simulink model "gm_hybrid_lht"  (R2019b)
settings: Solver=FixedStepDiscrete  StartTime=0.0  StopTime=inf  FixedStep=1/120e6  RelTol=1e-3
undefined symbols (not defined in the file or in its folder): bt, height, nTheta, width
libraries: hdlsllib x237, simulink x149, hdlmdlgenlib x11, dspsrcs4 x1
(part 6 of 11)

== system gm_hybrid_lht/Hybrid LHT/Hybrid LHT Accumulator/Accumulator with Switches/Accumulator_instance10/Block RAM ==
  wr_data : Inport  OutDataTypeStr=fixdt(0, 36, 0)  PortDimensions=1  SampleTime=8.33333333333333e-09
  wr_addr : Inport  Port=2  OutDataTypeStr=fixdt(0, 9, 0)  PortDimensions=1  SampleTime=8.33333333333333e-09
  wr_en : Inport  Port=3  OutDataTypeStr=boolean  PortDimensions=1  SampleTime=8.33333333333333e-09
  rd_addr : Inport  Port=4  OutDataTypeStr=fixdt(0, 9, 0)  PortDimensions=1  SampleTime=8.33333333333333e-09
  Simple Dual Port RAM Generator : Subsystem  mask{b=double(36), d=double(400), b_hidden=double(36), d_hidden=double(400)}
      mask prompts: b "Data width:"; d "Depth:"
      mask init: same as gm_hybrid_lht/Hybrid LHT/Hybrid LHT Accumulator/Accumulator with Switches/Accumulator_instance1/Block RAM/Simple Dual Port RAM Generator
  rd_data : Outport
  wires:
  rd_addr/1 -> Simple Dual Port RAM Generator/4(rd_addr)
  wr_en/1 -> Simple Dual Port RAM Generator/3(wr_en)
  wr_addr/1 -> Simple Dual Port RAM Generator/2(wr_addr)
  wr_data/1 -> Simple Dual Port RAM Generator/1(wr_data)
  Simple Dual Port RAM Generator/1(rd_data) -> rd_data/1

== system gm_hybrid_lht/Hybrid LHT/Hybrid LHT Accumulator/Accumulator with Switches/Accumulator_instance11/Block RAM ==
  wr_data : Inport  OutDataTypeStr=fixdt(0, 36, 0)  PortDimensions=1  SampleTime=8.33333333333333e-09
  wr_addr : Inport  Port=2  OutDataTypeStr=fixdt(0, 9, 0)  PortDimensions=1  SampleTime=8.33333333333333e-09
  wr_en : Inport  Port=3  OutDataTypeStr=boolean  PortDimensions=1  SampleTime=8.33333333333333e-09
  rd_addr : Inport  Port=4  OutDataTypeStr=fixdt(0, 9, 0)  PortDimensions=1  SampleTime=8.33333333333333e-09
  Simple Dual Port RAM Generator : Subsystem  mask{b=double(36), d=double(400), b_hidden=double(36), d_hidden=double(400)}
      mask prompts: b "Data width:"; d "Depth:"
      mask init: same as gm_hybrid_lht/Hybrid LHT/Hybrid LHT Accumulator/Accumulator with Switches/Accumulator_instance1/Block RAM/Simple Dual Port RAM Generator
  rd_data : Outport
  wires:
  rd_addr/1 -> Simple Dual Port RAM Generator/4(rd_addr)
  wr_en/1 -> Simple Dual Port RAM Generator/3(wr_en)
  wr_addr/1 -> Simple Dual Port RAM Generator/2(wr_addr)
  wr_data/1 -> Simple Dual Port RAM Generator/1(wr_data)
  Simple Dual Port RAM Generator/1(rd_data) -> rd_data/1

== system gm_hybrid_lht/Hybrid LHT/Hybrid LHT Accumulator/Accumulator with Switches/Accumulator_instance12/Block RAM ==
  wr_data : Inport  OutDataTypeStr=fixdt(0, 36, 0)  PortDimensions=1  SampleTime=8.33333333333333e-09
  wr_addr : Inport  Port=2  OutDataTypeStr=fixdt(0, 9, 0)  PortDimensions=1  SampleTime=8.33333333333333e-09
  wr_en : Inport  Port=3  OutDataTypeStr=boolean  PortDimensions=1  SampleTime=8.33333333333333e-09
  rd_addr : Inport  Port=4  OutDataTypeStr=fixdt(0, 9, 0)  PortDimensions=1  SampleTime=8.33333333333333e-09
  Simple Dual Port RAM Generator : Subsystem  mask{b=double(36), d=double(400), b_hidden=double(36), d_hidden=double(400)}
      mask prompts: b "Data width:"; d "Depth:"
      mask init: same as gm_hybrid_lht/Hybrid LHT/Hybrid LHT Accumulator/Accumulator with Switches/Accumulator_instance1/Block RAM/Simple Dual Port RAM Generator
  rd_data : Outport
  wires:
  rd_addr/1 -> Simple Dual Port RAM Generator/4(rd_addr)
  wr_en/1 -> Simple Dual Port RAM Generator/3(wr_en)
  wr_addr/1 -> Simple Dual Port RAM Generator/2(wr_addr)
  wr_data/1 -> Simple Dual Port RAM Generator/1(wr_data)
  Simple Dual Port RAM Generator/1(rd_data) -> rd_data/1

== system gm_hybrid_lht/Hybrid LHT/Hybrid LHT Accumulator/Accumulator with Switches/Accumulator_instance13/Block RAM ==
  wr_data : Inport  OutDataTypeStr=fixdt(0, 36, 0)  PortDimensions=1  SampleTime=8.33333333333333e-09
  wr_addr : Inport  Port=2  OutDataTypeStr=fixdt(0, 9, 0)  PortDimensions=1  SampleTime=8.33333333333333e-09
  wr_en : Inport  Port=3  OutDataTypeStr=boolean  PortDimensions=1  SampleTime=8.33333333333333e-09
  rd_addr : Inport  Port=4  OutDataTypeStr=fixdt(0, 9, 0)  PortDimensions=1  SampleTime=8.33333333333333e-09
  Simple Dual Port RAM Generator : Subsystem  mask{b=double(36), d=double(400), b_hidden=double(36), d_hidden=double(400)}
      mask prompts: b "Data width:"; d "Depth:"
      mask init: same as gm_hybrid_lht/Hybrid LHT/Hybrid LHT Accumulator/Accumulator with Switches/Accumulator_instance1/Block RAM/Simple Dual Port RAM Generator
  rd_data : Outport
  wires:
  rd_addr/1 -> Simple Dual Port RAM Generator/4(rd_addr)
  wr_en/1 -> Simple Dual Port RAM Generator/3(wr_en)
  wr_addr/1 -> Simple Dual Port RAM Generator/2(wr_addr)
  wr_data/1 -> Simple Dual Port RAM Generator/1(wr_data)
  Simple Dual Port RAM Generator/1(rd_data) -> rd_data/1

== system gm_hybrid_lht/Hybrid LHT/Hybrid LHT Accumulator/Accumulator with Switches/Accumulator_instance14/Block RAM ==
  wr_data : Inport  OutDataTypeStr=fixdt(0, 36, 0)  PortDimensions=1  SampleTime=8.33333333333333e-09
  wr_addr : Inport  Port=2  OutDataTypeStr=fixdt(0, 9, 0)  PortDimensions=1  SampleTime=8.33333333333333e-09
  wr_en : Inport  Port=3  OutDataTypeStr=boolean  PortDimensions=1  SampleTime=8.33333333333333e-09
  rd_addr : Inport  Port=4  OutDataTypeStr=fixdt(0, 9, 0)  PortDimensions=1  SampleTime=8.33333333333333e-09
  Simple Dual Port RAM Generator : Subsystem  mask{b=double(36), d=double(400), b_hidden=double(36), d_hidden=double(400)}
      mask prompts: b "Data width:"; d "Depth:"
      mask init: same as gm_hybrid_lht/Hybrid LHT/Hybrid LHT Accumulator/Accumulator with Switches/Accumulator_instance1/Block RAM/Simple Dual Port RAM Generator
  rd_data : Outport
  wires:
  rd_addr/1 -> Simple Dual Port RAM Generator/4(rd_addr)
  wr_en/1 -> Simple Dual Port RAM Generator/3(wr_en)
  wr_addr/1 -> Simple Dual Port RAM Generator/2(wr_addr)
  wr_data/1 -> Simple Dual Port RAM Generator/1(wr_data)
  Simple Dual Port RAM Generator/1(rd_data) -> rd_data/1

== system gm_hybrid_lht/Hybrid LHT/Hybrid LHT Accumulator/Accumulator with Switches/Accumulator_instance15/Block RAM ==
  wr_data : Inport  OutDataTypeStr=fixdt(0, 36, 0)  PortDimensions=1  SampleTime=8.33333333333333e-09
  wr_addr : Inport  Port=2  OutDataTypeStr=fixdt(0, 9, 0)  PortDimensions=1  SampleTime=8.33333333333333e-09
  wr_en : Inport  Port=3  OutDataTypeStr=boolean  PortDimensions=1  SampleTime=8.33333333333333e-09
  rd_addr : Inport  Port=4  OutDataTypeStr=fixdt(0, 9, 0)  PortDimensions=1  SampleTime=8.33333333333333e-09
  Simple Dual Port RAM Generator : Subsystem  mask{b=double(36), d=double(400), b_hidden=double(36), d_hidden=double(400)}
      mask prompts: b "Data width:"; d "Depth:"
      mask init: same as gm_hybrid_lht/Hybrid LHT/Hybrid LHT Accumulator/Accumulator with Switches/Accumulator_instance1/Block RAM/Simple Dual Port RAM Generator
  rd_data : Outport
  wires:
  rd_addr/1 -> Simple Dual Port RAM Generator/4(rd_addr)
  wr_en/1 -> Simple Dual Port RAM Generator/3(wr_en)
  wr_addr/1 -> Simple Dual Port RAM Generator/2(wr_addr)
  wr_data/1 -> Simple Dual Port RAM Generator/1(wr_data)
  Simple Dual Port RAM Generator/1(rd_data) -> rd_data/1

== system gm_hybrid_lht/Hybrid LHT/Hybrid LHT Accumulator/Accumulator with Switches/Accumulator_instance16/Block RAM ==
  wr_data : Inport  OutDataTypeStr=fixdt(0, 36, 0)  PortDimensions=1  SampleTime=8.33333333333333e-09
  wr_addr : Inport  Port=2  OutDataTypeStr=fixdt(0, 9, 0)  PortDimensions=1  SampleTime=8.33333333333333e-09
  wr_en : Inport  Port=3  OutDataTypeStr=boolean  PortDimensions=1  SampleTime=8.33333333333333e-09
  rd_addr : Inport  Port=4  OutDataTypeStr=fixdt(0, 9, 0)  PortDimensions=1  SampleTime=8.33333333333333e-09
  Simple Dual Port RAM Generator : Subsystem  mask{b=double(36), d=double(400), b_hidden=double(36), d_hidden=double(400)}
      mask prompts: b "Data width:"; d "Depth:"
      mask init: same as gm_hybrid_lht/Hybrid LHT/Hybrid LHT Accumulator/Accumulator with Switches/Accumulator_instance1/Block RAM/Simple Dual Port RAM Generator
  rd_data : Outport
  wires:
  rd_addr/1 -> Simple Dual Port RAM Generator/4(rd_addr)
  wr_en/1 -> Simple Dual Port RAM Generator/3(wr_en)
  wr_addr/1 -> Simple Dual Port RAM Generator/2(wr_addr)
  wr_data/1 -> Simple Dual Port RAM Generator/1(wr_data)
  Simple Dual Port RAM Generator/1(rd_data) -> rd_data/1

== system gm_hybrid_lht/Hybrid LHT/Hybrid LHT Accumulator/Accumulator with Switches/Accumulator_instance17/Block RAM ==
  wr_data : Inport  OutDataTypeStr=fixdt(0, 36, 0)  PortDimensions=1  SampleTime=8.33333333333333e-09
  wr_addr : Inport  Port=2  OutDataTypeStr=fixdt(0, 9, 0)  PortDimensions=1  SampleTime=8.33333333333333e-09
  wr_en : Inport  Port=3  OutDataTypeStr=boolean  PortDimensions=1  SampleTime=8.33333333333333e-09
  rd_addr : Inport  Port=4  OutDataTypeStr=fixdt(0, 9, 0)  PortDimensions=1  SampleTime=8.33333333333333e-09
  Simple Dual Port RAM Generator : Subsystem  mask{b=double(36), d=double(400), b_hidden=double(36), d_hidden=double(400)}
      mask prompts: b "Data width:"; d "Depth:"
      mask init: same as gm_hybrid_lht/Hybrid LHT/Hybrid LHT Accumulator/Accumulator with Switches/Accumulator_instance1/Block RAM/Simple Dual Port RAM Generator
  rd_data : Outport
  wires:
  rd_addr/1 -> Simple Dual Port RAM Generator/4(rd_addr)
  wr_en/1 -> Simple Dual Port RAM Generator/3(wr_en)
  wr_addr/1 -> Simple Dual Port RAM Generator/2(wr_addr)
  wr_data/1 -> Simple Dual Port RAM Generator/1(wr_data)
  Simple Dual Port RAM Generator/1(rd_data) -> rd_data/1

== system gm_hybrid_lht/Hybrid LHT/Hybrid LHT Accumulator/Accumulator with Switches/Accumulator_instance18/Block RAM ==
  wr_data : Inport  OutDataTypeStr=fixdt(0, 36, 0)  PortDimensions=1  SampleTime=8.33333333333333e-09
  wr_addr : Inport  Port=2  OutDataTypeStr=fixdt(0, 9, 0)  PortDimensions=1  SampleTime=8.33333333333333e-09
  wr_en : Inport  Port=3  OutDataTypeStr=boolean  PortDimensions=1  SampleTime=8.33333333333333e-09
  rd_addr : Inport  Port=4  OutDataTypeStr=fixdt(0, 9, 0)  PortDimensions=1  SampleTime=8.33333333333333e-09
  Simple Dual Port RAM Generator : Subsystem  mask{b=double(36), d=double(400), b_hidden=double(36), d_hidden=double(400)}
      mask prompts: b "Data width:"; d "Depth:"
      mask init: same as gm_hybrid_lht/Hybrid LHT/Hybrid LHT Accumulator/Accumulator with Switches/Accumulator_instance1/Block RAM/Simple Dual Port RAM Generator
  rd_data : Outport
  wires:
  rd_addr/1 -> Simple Dual Port RAM Generator/4(rd_addr)
  wr_en/1 -> Simple Dual Port RAM Generator/3(wr_en)
  wr_addr/1 -> Simple Dual Port RAM Generator/2(wr_addr)
  wr_data/1 -> Simple Dual Port RAM Generator/1(wr_data)
  Simple Dual Port RAM Generator/1(rd_data) -> rd_data/1

== system gm_hybrid_lht/Hybrid LHT/Hybrid LHT Accumulator/Accumulator with Switches/Accumulator_instance19/Block RAM ==
  wr_data : Inport  OutDataTypeStr=fixdt(0, 36, 0)  PortDimensions=1  SampleTime=8.33333333333333e-09
  wr_addr : Inport  Port=2  OutDataTypeStr=fixdt(0, 9, 0)  PortDimensions=1  SampleTime=8.33333333333333e-09
  wr_en : Inport  Port=3  OutDataTypeStr=boolean  PortDimensions=1  SampleTime=8.33333333333333e-09
  rd_addr : Inport  Port=4  OutDataTypeStr=fixdt(0, 9, 0)  PortDimensions=1  SampleTime=8.33333333333333e-09
  Simple Dual Port RAM Generator : Subsystem  mask{b=double(36), d=double(400), b_hidden=double(36), d_hidden=double(400)}
      mask prompts: b "Data width:"; d "Depth:"
      mask init: same as gm_hybrid_lht/Hybrid LHT/Hybrid LHT Accumulator/Accumulator with Switches/Accumulator_instance1/Block RAM/Simple Dual Port RAM Generator
  rd_data : Outport
  wires:
  rd_addr/1 -> Simple Dual Port RAM Generator/4(rd_addr)
  wr_en/1 -> Simple Dual Port RAM Generator/3(wr_en)
  wr_addr/1 -> Simple Dual Port RAM Generator/2(wr_addr)
  wr_data/1 -> Simple Dual Port RAM Generator/1(wr_data)
  Simple Dual Port RAM Generator/1(rd_data) -> rd_data/1

== system gm_hybrid_lht/Hybrid LHT/Hybrid LHT Accumulator/Accumulator with Switches/Accumulator_instance2/Block RAM ==
  wr_data : Inport  OutDataTypeStr=fixdt(0, 36, 0)  PortDimensions=1  SampleTime=8.33333333333333e-09
  wr_addr : Inport  Port=2  OutDataTypeStr=fixdt(0, 9, 0)  PortDimensions=1  SampleTime=8.33333333333333e-09
  wr_en : Inport  Port=3  OutDataTypeStr=boolean  PortDimensions=1  SampleTime=8.33333333333333e-09
  rd_addr : Inport  Port=4  OutDataTypeStr=fixdt(0, 9, 0)  PortDimensions=1  SampleTime=8.33333333333333e-09
  Simple Dual Port RAM Generator : Subsystem  mask{b=double(36), d=double(400), b_hidden=double(36), d_hidden=double(400)}
      mask prompts: b "Data width:"; d "Depth:"
      mask init: same as gm_hybrid_lht/Hybrid LHT/Hybrid LHT Accumulator/Accumulator with Switches/Accumulator_instance1/Block RAM/Simple Dual Port RAM Generator
  rd_data : Outport
  wires:
  rd_addr/1 -> Simple Dual Port RAM Generator/4(rd_addr)
  wr_en/1 -> Simple Dual Port RAM Generator/3(wr_en)
  wr_addr/1 -> Simple Dual Port RAM Generator/2(wr_addr)
  wr_data/1 -> Simple Dual Port RAM Generator/1(wr_data)
  Simple Dual Port RAM Generator/1(rd_data) -> rd_data/1

== system gm_hybrid_lht/Hybrid LHT/Hybrid LHT Accumulator/Accumulator with Switches/Accumulator_instance20/Block RAM ==
  wr_data : Inport  OutDataTypeStr=fixdt(0, 36, 0)  PortDimensions=1  SampleTime=8.33333333333333e-09
  wr_addr : Inport  Port=2  OutDataTypeStr=fixdt(0, 9, 0)  PortDimensions=1  SampleTime=8.33333333333333e-09
  wr_en : Inport  Port=3  OutDataTypeStr=boolean  PortDimensions=1  SampleTime=8.33333333333333e-09
  rd_addr : Inport  Port=4  OutDataTypeStr=fixdt(0, 9, 0)  PortDimensions=1  SampleTime=8.33333333333333e-09
  Simple Dual Port RAM Generator : Subsystem  mask{b=double(36), d=double(400), b_hidden=double(36), d_hidden=double(400)}
      mask prompts: b "Data width:"; d "Depth:"
      mask init: same as gm_hybrid_lht/Hybrid LHT/Hybrid LHT Accumulator/Accumulator with Switches/Accumulator_instance1/Block RAM/Simple Dual Port RAM Generator
  rd_data : Outport
  wires:
  rd_addr/1 -> Simple Dual Port RAM Generator/4(rd_addr)
  wr_en/1 -> Simple Dual Port RAM Generator/3(wr_en)
  wr_addr/1 -> Simple Dual Port RAM Generator/2(wr_addr)
  wr_data/1 -> Simple Dual Port RAM Generator/1(wr_data)
  Simple Dual Port RAM Generator/1(rd_data) -> rd_data/1

== system gm_hybrid_lht/Hybrid LHT/Hybrid LHT Accumulator/Accumulator with Switches/Accumulator_instance21/Block RAM ==
  wr_data : Inport  OutDataTypeStr=fixdt(0, 36, 0)  PortDimensions=1  SampleTime=8.33333333333333e-09
  wr_addr : Inport  Port=2  OutDataTypeStr=fixdt(0, 9, 0)  PortDimensions=1  SampleTime=8.33333333333333e-09
  wr_en : Inport  Port=3  OutDataTypeStr=boolean  PortDimensions=1  SampleTime=8.33333333333333e-09
  rd_addr : Inport  Port=4  OutDataTypeStr=fixdt(0, 9, 0)  PortDimensions=1  SampleTime=8.33333333333333e-09
  Simple Dual Port RAM Generator : Subsystem  mask{b=double(36), d=double(400), b_hidden=double(36), d_hidden=double(400)}
      mask prompts: b "Data width:"; d "Depth:"
      mask init: same as gm_hybrid_lht/Hybrid LHT/Hybrid LHT Accumulator/Accumulator with Switches/Accumulator_instance1/Block RAM/Simple Dual Port RAM Generator
  rd_data : Outport
  wires:
  rd_addr/1 -> Simple Dual Port RAM Generator/4(rd_addr)
  wr_en/1 -> Simple Dual Port RAM Generator/3(wr_en)
  wr_addr/1 -> Simple Dual Port RAM Generator/2(wr_addr)
  wr_data/1 -> Simple Dual Port RAM Generator/1(wr_data)
  Simple Dual Port RAM Generator/1(rd_data) -> rd_data/1

== system gm_hybrid_lht/Hybrid LHT/Hybrid LHT Accumulator/Accumulator with Switches/Accumulator_instance22/Block RAM ==
  wr_data : Inport  OutDataTypeStr=fixdt(0, 36, 0)  PortDimensions=1  SampleTime=8.33333333333333e-09
  wr_addr : Inport  Port=2  OutDataTypeStr=fixdt(0, 9, 0)  PortDimensions=1  SampleTime=8.33333333333333e-09
  wr_en : Inport  Port=3  OutDataTypeStr=boolean  PortDimensions=1  SampleTime=8.33333333333333e-09
  rd_addr : Inport  Port=4  OutDataTypeStr=fixdt(0, 9, 0)  PortDimensions=1  SampleTime=8.33333333333333e-09
  Simple Dual Port RAM Generator : Subsystem  mask{b=double(36), d=double(400), b_hidden=double(36), d_hidden=double(400)}
      mask prompts: b "Data width:"; d "Depth:"
      mask init: same as gm_hybrid_lht/Hybrid LHT/Hybrid LHT Accumulator/Accumulator with Switches/Accumulator_instance1/Block RAM/Simple Dual Port RAM Generator
  rd_data : Outport
  wires:
  rd_addr/1 -> Simple Dual Port RAM Generator/4(rd_addr)
  wr_en/1 -> Simple Dual Port RAM Generator/3(wr_en)
  wr_addr/1 -> Simple Dual Port RAM Generator/2(wr_addr)
  wr_data/1 -> Simple Dual Port RAM Generator/1(wr_data)
  Simple Dual Port RAM Generator/1(rd_data) -> rd_data/1

== system gm_hybrid_lht/Hybrid LHT/Hybrid LHT Accumulator/Accumulator with Switches/Accumulator_instance23/Block RAM ==
  wr_data : Inport  OutDataTypeStr=fixdt(0, 36, 0)  PortDimensions=1  SampleTime=8.33333333333333e-09
  wr_addr : Inport  Port=2  OutDataTypeStr=fixdt(0, 9, 0)  PortDimensions=1  SampleTime=8.33333333333333e-09
  wr_en : Inport  Port=3  OutDataTypeStr=boolean  PortDimensions=1  SampleTime=8.33333333333333e-09
  rd_addr : Inport  Port=4  OutDataTypeStr=fixdt(0, 9, 0)  PortDimensions=1  SampleTime=8.33333333333333e-09
  Simple Dual Port RAM Generator : Subsystem  mask{b=double(36), d=double(400), b_hidden=double(36), d_hidden=double(400)}
      mask prompts: b "Data width:"; d "Depth:"
      mask init: same as gm_hybrid_lht/Hybrid LHT/Hybrid LHT Accumulator/Accumulator with Switches/Accumulator_instance1/Block RAM/Simple Dual Port RAM Generator
  rd_data : Outport
  wires:
  rd_addr/1 -> Simple Dual Port RAM Generator/4(rd_addr)
  wr_en/1 -> Simple Dual Port RAM Generator/3(wr_en)
  wr_addr/1 -> Simple Dual Port RAM Generator/2(wr_addr)
  wr_data/1 -> Simple Dual Port RAM Generator/1(wr_data)
  Simple Dual Port RAM Generator/1(rd_data) -> rd_data/1

== system gm_hybrid_lht/Hybrid LHT/Hybrid LHT Accumulator/Accumulator with Switches/Accumulator_instance24/Block RAM ==
  wr_data : Inport  OutDataTypeStr=fixdt(0, 36, 0)  PortDimensions=1  SampleTime=8.33333333333333e-09
  wr_addr : Inport  Port=2  OutDataTypeStr=fixdt(0, 9, 0)  PortDimensions=1  SampleTime=8.33333333333333e-09
  wr_en : Inport  Port=3  OutDataTypeStr=boolean  PortDimensions=1  SampleTime=8.33333333333333e-09
  rd_addr : Inport  Port=4  OutDataTypeStr=fixdt(0, 9, 0)  PortDimensions=1  SampleTime=8.33333333333333e-09
  Simple Dual Port RAM Generator : Subsystem  mask{b=double(36), d=double(400), b_hidden=double(36), d_hidden=double(400)}
      mask prompts: b "Data width:"; d "Depth:"
      mask init: same as gm_hybrid_lht/Hybrid LHT/Hybrid LHT Accumulator/Accumulator with Switches/Accumulator_instance1/Block RAM/Simple Dual Port RAM Generator
  rd_data : Outport
  wires:
  rd_addr/1 -> Simple Dual Port RAM Generator/4(rd_addr)
  wr_en/1 -> Simple Dual Port RAM Generator/3(wr_en)
  wr_addr/1 -> Simple Dual Port RAM Generator/2(wr_addr)
  wr_data/1 -> Simple Dual Port RAM Generator/1(wr_data)
  Simple Dual Port RAM Generator/1(rd_data) -> rd_data/1

== system gm_hybrid_lht/Hybrid LHT/Hybrid LHT Accumulator/Accumulator with Switches/Accumulator_instance25/Block RAM ==
  wr_data : Inport  OutDataTypeStr=fixdt(0, 36, 0)  PortDimensions=1  SampleTime=8.33333333333333e-09
  wr_addr : Inport  Port=2  OutDataTypeStr=fixdt(0, 9, 0)  PortDimensions=1  SampleTime=8.33333333333333e-09
  wr_en : Inport  Port=3  OutDataTypeStr=boolean  PortDimensions=1  SampleTime=8.33333333333333e-09
  rd_addr : Inport  Port=4  OutDataTypeStr=fixdt(0, 9, 0)  PortDimensions=1  SampleTime=8.33333333333333e-09
  Simple Dual Port RAM Generator : Subsystem  mask{b=double(36), d=double(400), b_hidden=double(36), d_hidden=double(400)}
      mask prompts: b "Data width:"; d "Depth:"
      mask init: same as gm_hybrid_lht/Hybrid LHT/Hybrid LHT Accumulator/Accumulator with Switches/Accumulator_instance1/Block RAM/Simple Dual Port RAM Generator
  rd_data : Outport
  wires:
  rd_addr/1 -> Simple Dual Port RAM Generator/4(rd_addr)
  wr_en/1 -> Simple Dual Port RAM Generator/3(wr_en)
  wr_addr/1 -> Simple Dual Port RAM Generator/2(wr_addr)
  wr_data/1 -> Simple Dual Port RAM Generator/1(wr_data)
  Simple Dual Port RAM Generator/1(rd_data) -> rd_data/1

== system gm_hybrid_lht/Hybrid LHT/Hybrid LHT Accumulator/Accumulator with Switches/Accumulator_instance26/Block RAM ==
  wr_data : Inport  OutDataTypeStr=fixdt(0, 36, 0)  PortDimensions=1  SampleTime=8.33333333333333e-09
  wr_addr : Inport  Port=2  OutDataTypeStr=fixdt(0, 9, 0)  PortDimensions=1  SampleTime=8.33333333333333e-09
  wr_en : Inport  Port=3  OutDataTypeStr=boolean  PortDimensions=1  SampleTime=8.33333333333333e-09
  rd_addr : Inport  Port=4  OutDataTypeStr=fixdt(0, 9, 0)  PortDimensions=1  SampleTime=8.33333333333333e-09
  Simple Dual Port RAM Generator : Subsystem  mask{b=double(36), d=double(400), b_hidden=double(36), d_hidden=double(400)}
      mask prompts: b "Data width:"; d "Depth:"
      mask init: same as gm_hybrid_lht/Hybrid LHT/Hybrid LHT Accumulator/Accumulator with Switches/Accumulator_instance1/Block RAM/Simple Dual Port RAM Generator
  rd_data : Outport
  wires:
  rd_addr/1 -> Simple Dual Port RAM Generator/4(rd_addr)
  wr_en/1 -> Simple Dual Port RAM Generator/3(wr_en)
  wr_addr/1 -> Simple Dual Port RAM Generator/2(wr_addr)
  wr_data/1 -> Simple Dual Port RAM Generator/1(wr_data)
  Simple Dual Port RAM Generator/1(rd_data) -> rd_data/1

== system gm_hybrid_lht/Hybrid LHT/Hybrid LHT Accumulator/Accumulator with Switches/Accumulator_instance27/Block RAM ==
  wr_data : Inport  OutDataTypeStr=fixdt(0, 36, 0)  PortDimensions=1  SampleTime=8.33333333333333e-09
  wr_addr : Inport  Port=2  OutDataTypeStr=fixdt(0, 9, 0)  PortDimensions=1  SampleTime=8.33333333333333e-09
  wr_en : Inport  Port=3  OutDataTypeStr=boolean  PortDimensions=1  SampleTime=8.33333333333333e-09
  rd_addr : Inport  Port=4  OutDataTypeStr=fixdt(0, 9, 0)  PortDimensions=1  SampleTime=8.33333333333333e-09
  Simple Dual Port RAM Generator : Subsystem  mask{b=double(36), d=double(400), b_hidden=double(36), d_hidden=double(400)}
      mask prompts: b "Data width:"; d "Depth:"
      mask init: same as gm_hybrid_lht/Hybrid LHT/Hybrid LHT Accumulator/Accumulator with Switches/Accumulator_instance1/Block RAM/Simple Dual Port RAM Generator
  rd_data : Outport
  wires:
  rd_addr/1 -> Simple Dual Port RAM Generator/4(rd_addr)
  wr_en/1 -> Simple Dual Port RAM Generator/3(wr_en)
  wr_addr/1 -> Simple Dual Port RAM Generator/2(wr_addr)
  wr_data/1 -> Simple Dual Port RAM Generator/1(wr_data)
  Simple Dual Port RAM Generator/1(rd_data) -> rd_data/1

== system gm_hybrid_lht/Hybrid LHT/Hybrid LHT Accumulator/Accumulator with Switches/Accumulator_instance28/Block RAM ==
  wr_data : Inport  OutDataTypeStr=fixdt(0, 36, 0)  PortDimensions=1  SampleTime=8.33333333333333e-09
  wr_addr : Inport  Port=2  OutDataTypeStr=fixdt(0, 9, 0)  PortDimensions=1  SampleTime=8.33333333333333e-09
  wr_en : Inport  Port=3  OutDataTypeStr=boolean  PortDimensions=1  SampleTime=8.33333333333333e-09
  rd_addr : Inport  Port=4  OutDataTypeStr=fixdt(0, 9, 0)  PortDimensions=1  SampleTime=8.33333333333333e-09
  Simple Dual Port RAM Generator : Subsystem  mask{b=double(36), d=double(400), b_hidden=double(36), d_hidden=double(400)}
      mask prompts: b "Data width:"; d "Depth:"
      mask init: same as gm_hybrid_lht/Hybrid LHT/Hybrid LHT Accumulator/Accumulator with Switches/Accumulator_instance1/Block RAM/Simple Dual Port RAM Generator
  rd_data : Outport
  wires:
  rd_addr/1 -> Simple Dual Port RAM Generator/4(rd_addr)
  wr_en/1 -> Simple Dual Port RAM Generator/3(wr_en)
  wr_addr/1 -> Simple Dual Port RAM Generator/2(wr_addr)
  wr_data/1 -> Simple Dual Port RAM Generator/1(wr_data)
  Simple Dual Port RAM Generator/1(rd_data) -> rd_data/1

== system gm_hybrid_lht/Hybrid LHT/Hybrid LHT Accumulator/Accumulator with Switches/Accumulator_instance29/Block RAM ==
  wr_data : Inport  OutDataTypeStr=fixdt(0, 36, 0)  PortDimensions=1  SampleTime=8.33333333333333e-09
  wr_addr : Inport  Port=2  OutDataTypeStr=fixdt(0, 9, 0)  PortDimensions=1  SampleTime=8.33333333333333e-09
  wr_en : Inport  Port=3  OutDataTypeStr=boolean  PortDimensions=1  SampleTime=8.33333333333333e-09
  rd_addr : Inport  Port=4  OutDataTypeStr=fixdt(0, 9, 0)  PortDimensions=1  SampleTime=8.33333333333333e-09
  Simple Dual Port RAM Generator : Subsystem  mask{b=double(36), d=double(400), b_hidden=double(36), d_hidden=double(400)}
      mask prompts: b "Data width:"; d "Depth:"
      mask init: same as gm_hybrid_lht/Hybrid LHT/Hybrid LHT Accumulator/Accumulator with Switches/Accumulator_instance1/Block RAM/Simple Dual Port RAM Generator
  rd_data : Outport
  wires:
  rd_addr/1 -> Simple Dual Port RAM Generator/4(rd_addr)
  wr_en/1 -> Simple Dual Port RAM Generator/3(wr_en)
  wr_addr/1 -> Simple Dual Port RAM Generator/2(wr_addr)
  wr_data/1 -> Simple Dual Port RAM Generator/1(wr_data)
  Simple Dual Port RAM Generator/1(rd_data) -> rd_data/1

== system gm_hybrid_lht/Hybrid LHT/Hybrid LHT Accumulator/Accumulator with Switches/Accumulator_instance3/Block RAM ==
  wr_data : Inport  OutDataTypeStr=fixdt(0, 36, 0)  PortDimensions=1  SampleTime=8.33333333333333e-09
  wr_addr : Inport  Port=2  OutDataTypeStr=fixdt(0, 9, 0)  PortDimensions=1  SampleTime=8.33333333333333e-09
  wr_en : Inport  Port=3  OutDataTypeStr=boolean  PortDimensions=1  SampleTime=8.33333333333333e-09
  rd_addr : Inport  Port=4  OutDataTypeStr=fixdt(0, 9, 0)  PortDimensions=1  SampleTime=8.33333333333333e-09
  Simple Dual Port RAM Generator : Subsystem  mask{b=double(36), d=double(400), b_hidden=double(36), d_hidden=double(400)}
      mask prompts: b "Data width:"; d "Depth:"
      mask init: same as gm_hybrid_lht/Hybrid LHT/Hybrid LHT Accumulator/Accumulator with Switches/Accumulator_instance1/Block RAM/Simple Dual Port RAM Generator
  rd_data : Outport
  wires:
  rd_addr/1 -> Simple Dual Port RAM Generator/4(rd_addr)
  wr_en/1 -> Simple Dual Port RAM Generator/3(wr_en)
  wr_addr/1 -> Simple Dual Port RAM Generator/2(wr_addr)
  wr_data/1 -> Simple Dual Port RAM Generator/1(wr_data)
  Simple Dual Port RAM Generator/1(rd_data) -> rd_data/1

== system gm_hybrid_lht/Hybrid LHT/Hybrid LHT Accumulator/Accumulator with Switches/Accumulator_instance30/Block RAM ==
  wr_data : Inport  OutDataTypeStr=fixdt(0, 36, 0)  PortDimensions=1  SampleTime=8.33333333333333e-09
  wr_addr : Inport  Port=2  OutDataTypeStr=fixdt(0, 9, 0)  PortDimensions=1  SampleTime=8.33333333333333e-09
  wr_en : Inport  Port=3  OutDataTypeStr=boolean  PortDimensions=1  SampleTime=8.33333333333333e-09
  rd_addr : Inport  Port=4  OutDataTypeStr=fixdt(0, 9, 0)  PortDimensions=1  SampleTime=8.33333333333333e-09
  Simple Dual Port RAM Generator : Subsystem  mask{b=double(36), d=double(400), b_hidden=double(36), d_hidden=double(400)}
      mask prompts: b "Data width:"; d "Depth:"
      mask init: same as gm_hybrid_lht/Hybrid LHT/Hybrid LHT Accumulator/Accumulator with Switches/Accumulator_instance1/Block RAM/Simple Dual Port RAM Generator
  rd_data : Outport
  wires:
  rd_addr/1 -> Simple Dual Port RAM Generator/4(rd_addr)
  wr_en/1 -> Simple Dual Port RAM Generator/3(wr_en)
  wr_addr/1 -> Simple Dual Port RAM Generator/2(wr_addr)
  wr_data/1 -> Simple Dual Port RAM Generator/1(wr_data)
  Simple Dual Port RAM Generator/1(rd_data) -> rd_data/1

== system gm_hybrid_lht/Hybrid LHT/Hybrid LHT Accumulator/Accumulator with Switches/Accumulator_instance31/Block RAM ==
  wr_data : Inport  OutDataTypeStr=fixdt(0, 36, 0)  PortDimensions=1  SampleTime=8.33333333333333e-09
  wr_addr : Inport  Port=2  OutDataTypeStr=fixdt(0, 9, 0)  PortDimensions=1  SampleTime=8.33333333333333e-09
  wr_en : Inport  Port=3  OutDataTypeStr=boolean  PortDimensions=1  SampleTime=8.33333333333333e-09
  rd_addr : Inport  Port=4  OutDataTypeStr=fixdt(0, 9, 0)  PortDimensions=1  SampleTime=8.33333333333333e-09
  Simple Dual Port RAM Generator : Subsystem  mask{b=double(36), d=double(400), b_hidden=double(36), d_hidden=double(400)}
      mask prompts: b "Data width:"; d "Depth:"
      mask init: same as gm_hybrid_lht/Hybrid LHT/Hybrid LHT Accumulator/Accumulator with Switches/Accumulator_instance1/Block RAM/Simple Dual Port RAM Generator
  rd_data : Outport
  wires:
  rd_addr/1 -> Simple Dual Port RAM Generator/4(rd_addr)
  wr_en/1 -> Simple Dual Port RAM Generator/3(wr_en)
  wr_addr/1 -> Simple Dual Port RAM Generator/2(wr_addr)
  wr_data/1 -> Simple Dual Port RAM Generator/1(wr_data)
  Simple Dual Port RAM Generator/1(rd_data) -> rd_data/1

== system gm_hybrid_lht/Hybrid LHT/Hybrid LHT Accumulator/Accumulator with Switches/Accumulator_instance32/Block RAM ==
  wr_data : Inport  OutDataTypeStr=fixdt(0, 36, 0)  PortDimensions=1  SampleTime=8.33333333333333e-09
  wr_addr : Inport  Port=2  OutDataTypeStr=fixdt(0, 9, 0)  PortDimensions=1  SampleTime=8.33333333333333e-09
  wr_en : Inport  Port=3  OutDataTypeStr=boolean  PortDimensions=1  SampleTime=8.33333333333333e-09
  rd_addr : Inport  Port=4  OutDataTypeStr=fixdt(0, 9, 0)  PortDimensions=1  SampleTime=8.33333333333333e-09
  Simple Dual Port RAM Generator : Subsystem  mask{b=double(36), d=double(400), b_hidden=double(36), d_hidden=double(400)}
      mask prompts: b "Data width:"; d "Depth:"
      mask init: same as gm_hybrid_lht/Hybrid LHT/Hybrid LHT Accumulator/Accumulator with Switches/Accumulator_instance1/Block RAM/Simple Dual Port RAM Generator
  rd_data : Outport
  wires:
  rd_addr/1 -> Simple Dual Port RAM Generator/4(rd_addr)
  wr_en/1 -> Simple Dual Port RAM Generator/3(wr_en)
  wr_addr/1 -> Simple Dual Port RAM Generator/2(wr_addr)
  wr_data/1 -> Simple Dual Port RAM Generator/1(wr_data)
  Simple Dual Port RAM Generator/1(rd_data) -> rd_data/1

== system gm_hybrid_lht/Hybrid LHT/Hybrid LHT Accumulator/Accumulator with Switches/Accumulator_instance33/Block RAM ==
  wr_data : Inport  OutDataTypeStr=fixdt(0, 36, 0)  PortDimensions=1  SampleTime=8.33333333333333e-09
  wr_addr : Inport  Port=2  OutDataTypeStr=fixdt(0, 9, 0)  PortDimensions=1  SampleTime=8.33333333333333e-09
  wr_en : Inport  Port=3  OutDataTypeStr=boolean  PortDimensions=1  SampleTime=8.33333333333333e-09
  rd_addr : Inport  Port=4  OutDataTypeStr=fixdt(0, 9, 0)  PortDimensions=1  SampleTime=8.33333333333333e-09
  Simple Dual Port RAM Generator : Subsystem  mask{b=double(36), d=double(400), b_hidden=double(36), d_hidden=double(400)}
      mask prompts: b "Data width:"; d "Depth:"
      mask init: same as gm_hybrid_lht/Hybrid LHT/Hybrid LHT Accumulator/Accumulator with Switches/Accumulator_instance1/Block RAM/Simple Dual Port RAM Generator
  rd_data : Outport
  wires:
  rd_addr/1 -> Simple Dual Port RAM Generator/4(rd_addr)
  wr_en/1 -> Simple Dual Port RAM Generator/3(wr_en)
  wr_addr/1 -> Simple Dual Port RAM Generator/2(wr_addr)
  wr_data/1 -> Simple Dual Port RAM Generator/1(wr_data)
  Simple Dual Port RAM Generator/1(rd_data) -> rd_data/1

== system gm_hybrid_lht/Hybrid LHT/Hybrid LHT Accumulator/Accumulator with Switches/Accumulator_instance34/Block RAM ==
  wr_data : Inport  OutDataTypeStr=fixdt(0, 36, 0)  PortDimensions=1  SampleTime=8.33333333333333e-09
  wr_addr : Inport  Port=2  OutDataTypeStr=fixdt(0, 9, 0)  PortDimensions=1  SampleTime=8.33333333333333e-09
  wr_en : Inport  Port=3  OutDataTypeStr=boolean  PortDimensions=1  SampleTime=8.33333333333333e-09
  rd_addr : Inport  Port=4  OutDataTypeStr=fixdt(0, 9, 0)  PortDimensions=1  SampleTime=8.33333333333333e-09
  Simple Dual Port RAM Generator : Subsystem  mask{b=double(36), d=double(400), b_hidden=double(36), d_hidden=double(400)}
      mask prompts: b "Data width:"; d "Depth:"
      mask init: same as gm_hybrid_lht/Hybrid LHT/Hybrid LHT Accumulator/Accumulator with Switches/Accumulator_instance1/Block RAM/Simple Dual Port RAM Generator
  rd_data : Outport
  wires:
  rd_addr/1 -> Simple Dual Port RAM Generator/4(rd_addr)
  wr_en/1 -> Simple Dual Port RAM Generator/3(wr_en)
  wr_addr/1 -> Simple Dual Port RAM Generator/2(wr_addr)
  wr_data/1 -> Simple Dual Port RAM Generator/1(wr_data)
  Simple Dual Port RAM Generator/1(rd_data) -> rd_data/1

== system gm_hybrid_lht/Hybrid LHT/Hybrid LHT Accumulator/Accumulator with Switches/Accumulator_instance35/Block RAM ==
  wr_data : Inport  OutDataTypeStr=fixdt(0, 36, 0)  PortDimensions=1  SampleTime=8.33333333333333e-09
  wr_addr : Inport  Port=2  OutDataTypeStr=fixdt(0, 9, 0)  PortDimensions=1  SampleTime=8.33333333333333e-09
  wr_en : Inport  Port=3  OutDataTypeStr=boolean  PortDimensions=1  SampleTime=8.33333333333333e-09
  rd_addr : Inport  Port=4  OutDataTypeStr=fixdt(0, 9, 0)  PortDimensions=1  SampleTime=8.33333333333333e-09
  Simple Dual Port RAM Generator : Subsystem  mask{b=double(36), d=double(400), b_hidden=double(36), d_hidden=double(400)}
      mask prompts: b "Data width:"; d "Depth:"
      mask init: same as gm_hybrid_lht/Hybrid LHT/Hybrid LHT Accumulator/Accumulator with Switches/Accumulator_instance1/Block RAM/Simple Dual Port RAM Generator
  rd_data : Outport
  wires:
  rd_addr/1 -> Simple Dual Port RAM Generator/4(rd_addr)
  wr_en/1 -> Simple Dual Port RAM Generator/3(wr_en)
  wr_addr/1 -> Simple Dual Port RAM Generator/2(wr_addr)
  wr_data/1 -> Simple Dual Port RAM Generator/1(wr_data)
  Simple Dual Port RAM Generator/1(rd_data) -> rd_data/1

== system gm_hybrid_lht/Hybrid LHT/Hybrid LHT Accumulator/Accumulator with Switches/Accumulator_instance36/Block RAM ==
  wr_data : Inport  OutDataTypeStr=fixdt(0, 36, 0)  PortDimensions=1  SampleTime=8.33333333333333e-09
  wr_addr : Inport  Port=2  OutDataTypeStr=fixdt(0, 9, 0)  PortDimensions=1  SampleTime=8.33333333333333e-09
  wr_en : Inport  Port=3  OutDataTypeStr=boolean  PortDimensions=1  SampleTime=8.33333333333333e-09
  rd_addr : Inport  Port=4  OutDataTypeStr=fixdt(0, 9, 0)  PortDimensions=1  SampleTime=8.33333333333333e-09
  Simple Dual Port RAM Generator : Subsystem  mask{b=double(36), d=double(400), b_hidden=double(36), d_hidden=double(400)}
      mask prompts: b "Data width:"; d "Depth:"
      mask init: same as gm_hybrid_lht/Hybrid LHT/Hybrid LHT Accumulator/Accumulator with Switches/Accumulator_instance1/Block RAM/Simple Dual Port RAM Generator
  rd_data : Outport
  wires:
  rd_addr/1 -> Simple Dual Port RAM Generator/4(rd_addr)
  wr_en/1 -> Simple Dual Port RAM Generator/3(wr_en)
  wr_addr/1 -> Simple Dual Port RAM Generator/2(wr_addr)
  wr_data/1 -> Simple Dual Port RAM Generator/1(wr_data)
  Simple Dual Port RAM Generator/1(rd_data) -> rd_data/1

== system gm_hybrid_lht/Hybrid LHT/Hybrid LHT Accumulator/Accumulator with Switches/Accumulator_instance37/Block RAM ==
  wr_data : Inport  OutDataTypeStr=fixdt(0, 36, 0)  PortDimensions=1  SampleTime=8.33333333333333e-09
  wr_addr : Inport  Port=2  OutDataTypeStr=fixdt(0, 9, 0)  PortDimensions=1  SampleTime=8.33333333333333e-09
  wr_en : Inport  Port=3  OutDataTypeStr=boolean  PortDimensions=1  SampleTime=8.33333333333333e-09
  rd_addr : Inport  Port=4  OutDataTypeStr=fixdt(0, 9, 0)  PortDimensions=1  SampleTime=8.33333333333333e-09
  Simple Dual Port RAM Generator : Subsystem  mask{b=double(36), d=double(400), b_hidden=double(36), d_hidden=double(400)}
      mask prompts: b "Data width:"; d "Depth:"
      mask init: same as gm_hybrid_lht/Hybrid LHT/Hybrid LHT Accumulator/Accumulator with Switches/Accumulator_instance1/Block RAM/Simple Dual Port RAM Generator
  rd_data : Outport
  wires:
  rd_addr/1 -> Simple Dual Port RAM Generator/4(rd_addr)
  wr_en/1 -> Simple Dual Port RAM Generator/3(wr_en)
  wr_addr/1 -> Simple Dual Port RAM Generator/2(wr_addr)
  wr_data/1 -> Simple Dual Port RAM Generator/1(wr_data)
  Simple Dual Port RAM Generator/1(rd_data) -> rd_data/1

== system gm_hybrid_lht/Hybrid LHT/Hybrid LHT Accumulator/Accumulator with Switches/Accumulator_instance38/Block RAM ==
  wr_data : Inport  OutDataTypeStr=fixdt(0, 36, 0)  PortDimensions=1  SampleTime=8.33333333333333e-09
  wr_addr : Inport  Port=2  OutDataTypeStr=fixdt(0, 9, 0)  PortDimensions=1  SampleTime=8.33333333333333e-09
  wr_en : Inport  Port=3  OutDataTypeStr=boolean  PortDimensions=1  SampleTime=8.33333333333333e-09
  rd_addr : Inport  Port=4  OutDataTypeStr=fixdt(0, 9, 0)  PortDimensions=1  SampleTime=8.33333333333333e-09
  Simple Dual Port RAM Generator : Subsystem  mask{b=double(36), d=double(400), b_hidden=double(36), d_hidden=double(400)}
      mask prompts: b "Data width:"; d "Depth:"
      mask init: same as gm_hybrid_lht/Hybrid LHT/Hybrid LHT Accumulator/Accumulator with Switches/Accumulator_instance1/Block RAM/Simple Dual Port RAM Generator
  rd_data : Outport
  wires:
  rd_addr/1 -> Simple Dual Port RAM Generator/4(rd_addr)
  wr_en/1 -> Simple Dual Port RAM Generator/3(wr_en)
  wr_addr/1 -> Simple Dual Port RAM Generator/2(wr_addr)
  wr_data/1 -> Simple Dual Port RAM Generator/1(wr_data)
  Simple Dual Port RAM Generator/1(rd_data) -> rd_data/1

== system gm_hybrid_lht/Hybrid LHT/Hybrid LHT Accumulator/Accumulator with Switches/Accumulator_instance39/Block RAM ==
  wr_data : Inport  OutDataTypeStr=fixdt(0, 36, 0)  PortDimensions=1  SampleTime=8.33333333333333e-09
  wr_addr : Inport  Port=2  OutDataTypeStr=fixdt(0, 9, 0)  PortDimensions=1  SampleTime=8.33333333333333e-09
  wr_en : Inport  Port=3  OutDataTypeStr=boolean  PortDimensions=1  SampleTime=8.33333333333333e-09
  rd_addr : Inport  Port=4  OutDataTypeStr=fixdt(0, 9, 0)  PortDimensions=1  SampleTime=8.33333333333333e-09
  Simple Dual Port RAM Generator : Subsystem  mask{b=double(36), d=double(400), b_hidden=double(36), d_hidden=double(400)}
      mask prompts: b "Data width:"; d "Depth:"
      mask init: same as gm_hybrid_lht/Hybrid LHT/Hybrid LHT Accumulator/Accumulator with Switches/Accumulator_instance1/Block RAM/Simple Dual Port RAM Generator
  rd_data : Outport
  wires:
  rd_addr/1 -> Simple Dual Port RAM Generator/4(rd_addr)
  wr_en/1 -> Simple Dual Port RAM Generator/3(wr_en)
  wr_addr/1 -> Simple Dual Port RAM Generator/2(wr_addr)
  wr_data/1 -> Simple Dual Port RAM Generator/1(wr_data)
  Simple Dual Port RAM Generator/1(rd_data) -> rd_data/1

== system gm_hybrid_lht/Hybrid LHT/Hybrid LHT Accumulator/Accumulator with Switches/Accumulator_instance4/Block RAM ==
  wr_data : Inport  OutDataTypeStr=fixdt(0, 36, 0)  PortDimensions=1  SampleTime=8.33333333333333e-09
  wr_addr : Inport  Port=2  OutDataTypeStr=fixdt(0, 9, 0)  PortDimensions=1  SampleTime=8.33333333333333e-09
  wr_en : Inport  Port=3  OutDataTypeStr=boolean  PortDimensions=1  SampleTime=8.33333333333333e-09
  rd_addr : Inport  Port=4  OutDataTypeStr=fixdt(0, 9, 0)  PortDimensions=1  SampleTime=8.33333333333333e-09
  Simple Dual Port RAM Generator : Subsystem  mask{b=double(36), d=double(400), b_hidden=double(36), d_hidden=double(400)}
      mask prompts: b "Data width:"; d "Depth:"
      mask init: same as gm_hybrid_lht/Hybrid LHT/Hybrid LHT Accumulator/Accumulator with Switches/Accumulator_instance1/Block RAM/Simple Dual Port RAM Generator
  rd_data : Outport
  wires:
  rd_addr/1 -> Simple Dual Port RAM Generator/4(rd_addr)
  wr_en/1 -> Simple Dual Port RAM Generator/3(wr_en)
  wr_addr/1 -> Simple Dual Port RAM Generator/2(wr_addr)
  wr_data/1 -> Simple Dual Port RAM Generator/1(wr_data)
  Simple Dual Port RAM Generator/1(rd_data) -> rd_data/1

== system gm_hybrid_lht/Hybrid LHT/Hybrid LHT Accumulator/Accumulator with Switches/Accumulator_instance40/Block RAM ==
  wr_data : Inport  OutDataTypeStr=fixdt(0, 36, 0)  PortDimensions=1  SampleTime=8.33333333333333e-09
  wr_addr : Inport  Port=2  OutDataTypeStr=fixdt(0, 9, 0)  PortDimensions=1  SampleTime=8.33333333333333e-09
  wr_en : Inport  Port=3  OutDataTypeStr=boolean  PortDimensions=1  SampleTime=8.33333333333333e-09
  rd_addr : Inport  Port=4  OutDataTypeStr=fixdt(0, 9, 0)  PortDimensions=1  SampleTime=8.33333333333333e-09
  Simple Dual Port RAM Generator : Subsystem  mask{b=double(36), d=double(400), b_hidden=double(36), d_hidden=double(400)}
      mask prompts: b "Data width:"; d "Depth:"
      mask init: same as gm_hybrid_lht/Hybrid LHT/Hybrid LHT Accumulator/Accumulator with Switches/Accumulator_instance1/Block RAM/Simple Dual Port RAM Generator
  rd_data : Outport
  wires:
  rd_addr/1 -> Simple Dual Port RAM Generator/4(rd_addr)
  wr_en/1 -> Simple Dual Port RAM Generator/3(wr_en)
  wr_addr/1 -> Simple Dual Port RAM Generator/2(wr_addr)
  wr_data/1 -> Simple Dual Port RAM Generator/1(wr_data)
  Simple Dual Port RAM Generator/1(rd_data) -> rd_data/1

== system gm_hybrid_lht/Hybrid LHT/Hybrid LHT Accumulator/Accumulator with Switches/Accumulator_instance41/Block RAM ==
  wr_data : Inport  OutDataTypeStr=fixdt(0, 36, 0)  PortDimensions=1  SampleTime=8.33333333333333e-09
  wr_addr : Inport  Port=2  OutDataTypeStr=fixdt(0, 9, 0)  PortDimensions=1  SampleTime=8.33333333333333e-09
  wr_en : Inport  Port=3  OutDataTypeStr=boolean  PortDimensions=1  SampleTime=8.33333333333333e-09
  rd_addr : Inport  Port=4  OutDataTypeStr=fixdt(0, 9, 0)  PortDimensions=1  SampleTime=8.33333333333333e-09
  Simple Dual Port RAM Generator : Subsystem  mask{b=double(36), d=double(400), b_hidden=double(36), d_hidden=double(400)}
      mask prompts: b "Data width:"; d "Depth:"
      mask init: same as gm_hybrid_lht/Hybrid LHT/Hybrid LHT Accumulator/Accumulator with Switches/Accumulator_instance1/Block RAM/Simple Dual Port RAM Generator
  rd_data : Outport
  wires:
  rd_addr/1 -> Simple Dual Port RAM Generator/4(rd_addr)
  wr_en/1 -> Simple Dual Port RAM Generator/3(wr_en)
  wr_addr/1 -> Simple Dual Port RAM Generator/2(wr_addr)
  wr_data/1 -> Simple Dual Port RAM Generator/1(wr_data)
  Simple Dual Port RAM Generator/1(rd_data) -> rd_data/1

== system gm_hybrid_lht/Hybrid LHT/Hybrid LHT Accumulator/Accumulator with Switches/Accumulator_instance42/Block RAM ==
  wr_data : Inport  OutDataTypeStr=fixdt(0, 36, 0)  PortDimensions=1  SampleTime=8.33333333333333e-09
  wr_addr : Inport  Port=2  OutDataTypeStr=fixdt(0, 9, 0)  PortDimensions=1  SampleTime=8.33333333333333e-09
  wr_en : Inport  Port=3  OutDataTypeStr=boolean  PortDimensions=1  SampleTime=8.33333333333333e-09
  rd_addr : Inport  Port=4  OutDataTypeStr=fixdt(0, 9, 0)  PortDimensions=1  SampleTime=8.33333333333333e-09
  Simple Dual Port RAM Generator : Subsystem  mask{b=double(36), d=double(400), b_hidden=double(36), d_hidden=double(400)}
      mask prompts: b "Data width:"; d "Depth:"
      mask init: same as gm_hybrid_lht/Hybrid LHT/Hybrid LHT Accumulator/Accumulator with Switches/Accumulator_instance1/Block RAM/Simple Dual Port RAM Generator
  rd_data : Outport
  wires:
  rd_addr/1 -> Simple Dual Port RAM Generator/4(rd_addr)
  wr_en/1 -> Simple Dual Port RAM Generator/3(wr_en)
  wr_addr/1 -> Simple Dual Port RAM Generator/2(wr_addr)
  wr_data/1 -> Simple Dual Port RAM Generator/1(wr_data)
  Simple Dual Port RAM Generator/1(rd_data) -> rd_data/1

== system gm_hybrid_lht/Hybrid LHT/Hybrid LHT Accumulator/Accumulator with Switches/Accumulator_instance43/Block RAM ==
  wr_data : Inport  OutDataTypeStr=fixdt(0, 36, 0)  PortDimensions=1  SampleTime=8.33333333333333e-09
  wr_addr : Inport  Port=2  OutDataTypeStr=fixdt(0, 9, 0)  PortDimensions=1  SampleTime=8.33333333333333e-09
  wr_en : Inport  Port=3  OutDataTypeStr=boolean  PortDimensions=1  SampleTime=8.33333333333333e-09
  rd_addr : Inport  Port=4  OutDataTypeStr=fixdt(0, 9, 0)  PortDimensions=1  SampleTime=8.33333333333333e-09
  Simple Dual Port RAM Generator : Subsystem  mask{b=double(36), d=double(400), b_hidden=double(36), d_hidden=double(400)}
      mask prompts: b "Data width:"; d "Depth:"
      mask init: same as gm_hybrid_lht/Hybrid LHT/Hybrid LHT Accumulator/Accumulator with Switches/Accumulator_instance1/Block RAM/Simple Dual Port RAM Generator
  rd_data : Outport
  wires:
  rd_addr/1 -> Simple Dual Port RAM Generator/4(rd_addr)
  wr_en/1 -> Simple Dual Port RAM Generator/3(wr_en)
  wr_addr/1 -> Simple Dual Port RAM Generator/2(wr_addr)
  wr_data/1 -> Simple Dual Port RAM Generator/1(wr_data)
  Simple Dual Port RAM Generator/1(rd_data) -> rd_data/1

== system gm_hybrid_lht/Hybrid LHT/Hybrid LHT Accumulator/Accumulator with Switches/Accumulator_instance44/Block RAM ==
  wr_data : Inport  OutDataTypeStr=fixdt(0, 36, 0)  PortDimensions=1  SampleTime=8.33333333333333e-09
  wr_addr : Inport  Port=2  OutDataTypeStr=fixdt(0, 9, 0)  PortDimensions=1  SampleTime=8.33333333333333e-09
  wr_en : Inport  Port=3  OutDataTypeStr=boolean  PortDimensions=1  SampleTime=8.33333333333333e-09
  rd_addr : Inport  Port=4  OutDataTypeStr=fixdt(0, 9, 0)  PortDimensions=1  SampleTime=8.33333333333333e-09
  Simple Dual Port RAM Generator : Subsystem  mask{b=double(36), d=double(400), b_hidden=double(36), d_hidden=double(400)}
      mask prompts: b "Data width:"; d "Depth:"
      mask init: same as gm_hybrid_lht/Hybrid LHT/Hybrid LHT Accumulator/Accumulator with Switches/Accumulator_instance1/Block RAM/Simple Dual Port RAM Generator
  rd_data : Outport
  wires:
  rd_addr/1 -> Simple Dual Port RAM Generator/4(rd_addr)
  wr_en/1 -> Simple Dual Port RAM Generator/3(wr_en)
  wr_addr/1 -> Simple Dual Port RAM Generator/2(wr_addr)
  wr_data/1 -> Simple Dual Port RAM Generator/1(wr_data)
  Simple Dual Port RAM Generator/1(rd_data) -> rd_data/1

== system gm_hybrid_lht/Hybrid LHT/Hybrid LHT Accumulator/Accumulator with Switches/Accumulator_instance45/Block RAM ==
  wr_data : Inport  OutDataTypeStr=fixdt(0, 36, 0)  PortDimensions=1  SampleTime=8.33333333333333e-09
  wr_addr : Inport  Port=2  OutDataTypeStr=fixdt(0, 9, 0)  PortDimensions=1  SampleTime=8.33333333333333e-09
  wr_en : Inport  Port=3  OutDataTypeStr=boolean  PortDimensions=1  SampleTime=8.33333333333333e-09
  rd_addr : Inport  Port=4  OutDataTypeStr=fixdt(0, 9, 0)  PortDimensions=1  SampleTime=8.33333333333333e-09
  Simple Dual Port RAM Generator : Subsystem  mask{b=double(36), d=double(400), b_hidden=double(36), d_hidden=double(400)}
      mask prompts: b "Data width:"; d "Depth:"
      mask init: same as gm_hybrid_lht/Hybrid LHT/Hybrid LHT Accumulator/Accumulator with Switches/Accumulator_instance1/Block RAM/Simple Dual Port RAM Generator
  rd_data : Outport
  wires:
  rd_addr/1 -> Simple Dual Port RAM Generator/4(rd_addr)
  wr_en/1 -> Simple Dual Port RAM Generator/3(wr_en)
  wr_addr/1 -> Simple Dual Port RAM Generator/2(wr_addr)
  wr_data/1 -> Simple Dual Port RAM Generator/1(wr_data)
  Simple Dual Port RAM Generator/1(rd_data) -> rd_data/1

== system gm_hybrid_lht/Hybrid LHT/Hybrid LHT Accumulator/Accumulator with Switches/Accumulator_instance5/Block RAM ==
  wr_data : Inport  OutDataTypeStr=fixdt(0, 36, 0)  PortDimensions=1  SampleTime=8.33333333333333e-09
  wr_addr : Inport  Port=2  OutDataTypeStr=fixdt(0, 9, 0)  PortDimensions=1  SampleTime=8.33333333333333e-09
  wr_en : Inport  Port=3  OutDataTypeStr=boolean  PortDimensions=1  SampleTime=8.33333333333333e-09
  rd_addr : Inport  Port=4  OutDataTypeStr=fixdt(0, 9, 0)  PortDimensions=1  SampleTime=8.33333333333333e-09
  Simple Dual Port RAM Generator : Subsystem  mask{b=double(36), d=double(400), b_hidden=double(36), d_hidden=double(400)}
      mask prompts: b "Data width:"; d "Depth:"
      mask init: same as gm_hybrid_lht/Hybrid LHT/Hybrid LHT Accumulator/Accumulator with Switches/Accumulator_instance1/Block RAM/Simple Dual Port RAM Generator
  rd_data : Outport
  wires:
  rd_addr/1 -> Simple Dual Port RAM Generator/4(rd_addr)
  wr_en/1 -> Simple Dual Port RAM Generator/3(wr_en)
  wr_addr/1 -> Simple Dual Port RAM Generator/2(wr_addr)
  wr_data/1 -> Simple Dual Port RAM Generator/1(wr_data)
  Simple Dual Port RAM Generator/1(rd_data) -> rd_data/1

== system gm_hybrid_lht/Hybrid LHT/Hybrid LHT Accumulator/Accumulator with Switches/Accumulator_instance6/Block RAM ==
  wr_data : Inport  OutDataTypeStr=fixdt(0, 36, 0)  PortDimensions=1  SampleTime=8.33333333333333e-09
  wr_addr : Inport  Port=2  OutDataTypeStr=fixdt(0, 9, 0)  PortDimensions=1  SampleTime=8.33333333333333e-09
  wr_en : Inport  Port=3  OutDataTypeStr=boolean  PortDimensions=1  SampleTime=8.33333333333333e-09
  rd_addr : Inport  Port=4  OutDataTypeStr=fixdt(0, 9, 0)  PortDimensions=1  SampleTime=8.33333333333333e-09
  Simple Dual Port RAM Generator : Subsystem  mask{b=double(36), d=double(400), b_hidden=double(36), d_hidden=double(400)}
      mask prompts: b "Data width:"; d "Depth:"
      mask init: same as gm_hybrid_lht/Hybrid LHT/Hybrid LHT Accumulator/Accumulator with Switches/Accumulator_instance1/Block RAM/Simple Dual Port RAM Generator
  rd_data : Outport
  wires:
  rd_addr/1 -> Simple Dual Port RAM Generator/4(rd_addr)
  wr_en/1 -> Simple Dual Port RAM Generator/3(wr_en)
  wr_addr/1 -> Simple Dual Port RAM Generator/2(wr_addr)
  wr_data/1 -> Simple Dual Port RAM Generator/1(wr_data)
  Simple Dual Port RAM Generator/1(rd_data) -> rd_data/1
